simulink model "jellystone_v4"  (R2016b)
settings: Solver=VariableStepAuto  StartTime=0.0  StopTime=30  RelTol=1e-3
values from neighbouring files (symbols this model uses):
  C0 = 2.017+(rand-.5)*.404    [executeModel.m]    (also in project.m)
  E0 = 31.217+(rand-.5)*6.244    [executeModel.m]    (also in project.m)
  W0 = 0    [executeModel.m]    (also in project.m)
settings Model: Creator=thomaskennedy  LastModifiedBy=thomaskennedy
settings DebuggingCC: InitInArrayFormatMsg=none

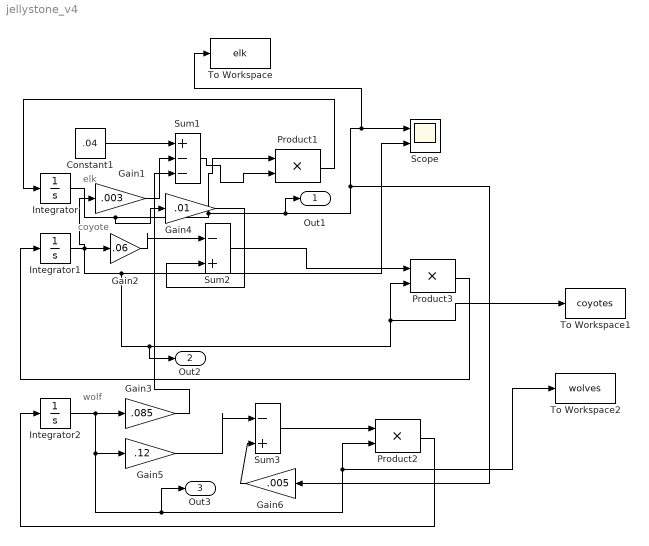
== system jellystone_v4 ==
  note: elk
  note: coyote
  note: wolf
  Constant1 : Constant  Value=.04
  Gain1 : Gain  Gain=.003  SaturateOnIntegerOverflow=on  OutDataTypeStr=Inherit: Same as input  ParamDataTypeStr=Inherit: Same as input
  Gain2 : Gain  Gain=.06  SaturateOnIntegerOverflow=on  OutDataTypeStr=Inherit: Same as input  ParamDataTypeStr=Inherit: Same as input
  Gain3 : Gain  Gain=.085  SaturateOnIntegerOverflow=on  OutDataTypeStr=Inherit: Same as input  ParamDataTypeStr=Inherit: Same as input
  Gain4 : Gain  Gain=.01  SaturateOnIntegerOverflow=on  OutDataTypeStr=Inherit: Same as input  ParamDataTypeStr=Inherit: Same as input
  Gain5 : Gain  Gain=.12  SaturateOnIntegerOverflow=on  OutDataTypeStr=Inherit: Same as input  ParamDataTypeStr=Inherit: Same as input
  Gain6 : Gain  Gain=.005  SaturateOnIntegerOverflow=on  OutDataTypeStr=Inherit: Same as input  ParamDataTypeStr=Inherit: Same as input
  Integrator : Integrator  InitialCondition=E0
  Integrator1 : Integrator  InitialCondition=C0
  Integrator2 : Integrator  InitialCondition=W0
  Product1 : Product  SaturateOnIntegerOverflow=on  InputSameDT=on  OutDataTypeStr=Inherit: Same as first input
  Product2 : Product  SaturateOnIntegerOverflow=on  InputSameDT=on  OutDataTypeStr=Inherit: Same as first input
  Product3 : Product  SaturateOnIntegerOverflow=on  InputSameDT=on  OutDataTypeStr=Inherit: Same as first input
  Scope : Scope  NumInputPorts=2
  Sum1 : Sum  Inputs=|+||-||-|  SaturateOnIntegerOverflow=on  InputSameDT=on  OutDataTypeStr=Inherit: Same as first input
  Sum2 : Sum  Inputs=|-||+|  SaturateOnIntegerOverflow=on  InputSameDT=on  OutDataTypeStr=Inherit: Same as first input
  Sum3 : Sum  Inputs=|-||+|  SaturateOnIntegerOverflow=on  InputSameDT=on  OutDataTypeStr=Inherit: Same as first input
  To Workspace : ToWorkspace  VariableName=elk  SampleTime=-1
  To Workspace1 : ToWorkspace  VariableName=coyotes  SampleTime=-1
  To Workspace2 : ToWorkspace  VariableName=wolves  SampleTime=-1
  Out1 : Outport
  Out2 : Outport  Port=2
  Out3 : Outport  Port=3
  wires:
  Constant1/1 -> Sum1/1
  Integrator1/1 -> Gain2/1, Out2/1, To Workspace1/1, Product3/2, Scope/2, Gain1/1
  Integrator/1 -> Gain4/1, Out1/1, Gain6/1, Scope/1, To Workspace/1, Product1/1
  Product1/1 -> Integrator/1
  Sum2/1 -> Product3/1
  Product3/1 -> Integrator1/1
  Sum1/1 -> Product1/2
  Gain1/1 -> Sum1/2
  Integrator2/1 -> Out3/1, To Workspace2/1, Product2/2, Gain5/1, Gain3/1
  Gain3/1 -> Sum1/3
  Gain2/1 -> Sum2/1
  Gain4/1 -> Sum2/2
  Gain5/1 -> Sum3/1
  Gain6/1 -> Sum3/2
  Sum3/1 -> Product2/1
  Product2/1 -> Integrator2/1
